simulink model "Full_Model_D_R6"  (R2013a)
settings: Solver=ode45  StartTime=0.0  StopTime=sim_length  MaxStep=1e-4  RelTol=1e-3
values from neighbouring files (symbols this model uses):
  A_Height_d = [1  0.02  0.00306066709295; 0  1  0.292172619905; 0  0  0.751477293075]    [Height_Controller_SS_D_Data.mat]    (also in Height_Controller_Sample_Time.m = A_d)
  A_Roll_d = [1  0.02  0.00957373027909; 0  1  0.913912481482; 0  0  0.751477293075]    [Roll_Controller_SS_D_Data.mat]    (also in Roll_Controller_Sample_Time.m = A_d)
  A_x_d = [1  0.725237004499; 0  0.506103765926]    [xy_Controller_PD_D_Data.mat]    (also in xy_Controller_PID_D_Data.mat; xy_Controller_Sample_Time.m = sys_d.a; xy_Controller_Sample_Time_2.m = sys_d.a)
  A_Yaw_d = [1  0.02  0.000714353321797; 0  1  0.0681924806681; 0  0  0.751477293075]    [Yaw_Controller_SS_D_Data.mat]    (also in Yaw_Controller_Sample_Time.m = A_d)
  B_Height_d = [0.000298297262238 0.0437238156136 0.248522706925]    [Height_Controller_SS_D_Data.mat]    (also in Height_Controller_Sample_Time.m = B_d)
  B_Roll_d = [0.000933070289885 0.136767575416 0.248522706925]    [Roll_Controller_SS_D_Data.mat]    (also in Roll_Controller_Sample_Time.m = B_d)
  B_x_d = [3.95796081795 7.11457501414]    [xy_Controller_PD_D_Data.mat]    (also in xy_Controller_PID_D_Data.mat; xy_Controller_Sample_Time.m = sys_d.b; xy_Controller_Sample_Time_2.m = sys_d.b)
  B_Yaw_d = [7.15569400366e-05 0.0103985455153 0.248522706925]    [Yaw_Controller_SS_D_Data.mat]    (also in Yaw_Controller_Sample_Time.m = B_d)
  C_Height_d = [1 0 0]    [Height_Controller_SS_D_Data.mat]    (also in Height_Controller_Sample_Time.m = C_d)
  C_Roll_d = [1  0  0; 0  1  0]    [Roll_Controller_SS_D_Data.mat]    (also in Roll_Controller_Sample_Time.m = C_d)
  C_x_d = [1 0]    [xy_Controller_PD_D_Data.mat]    (also in xy_Controller_PID_D_Data.mat; xy_Controller_Sample_Time.m = sys_d.c; xy_Controller_Sample_Time_2.m = sys_d.c)
  C_Yaw_d = [1  0  0; 0  1  0]    [Yaw_Controller_SS_D_Data.mat]    (also in Yaw_Controller_Sample_Time.m = C_d)
  coeff_speed1 = [-597.852411164 15567.4958959 -112629.522245 385376.825444 -722286.582234 762343.511164 -424427.181206 96698.0914793]    [Model_Parameters.mat]
  coeff_speed2 = [-33137.8630803 359389.817861 -1655728.0128 4197976.53355 -6322358.45977 5652250.74311 -2774846.33743 576528.840344]    [Model_Parameters.mat]
  coeff_speed3 = [-11936.4686056 137218.314774 -666283.661319 1770733.67902 -2780453.20018 2577948.57948 -1305141.01347 277978.291866]    [Model_Parameters.mat]
  coeff_speed4 = [-6669.45808334 79913.0612752 -401123.444791 1094619.31774 -1754742.75761 1652252.04897 -844945.337957 180729.993964]    [Model_Parameters.mat]
  coeff_thrust1 = [411.996230985 -4101.92524784 17203.3662669 -39329.1303747 52812.747408 -41528.8245566 17635.526271 -3103.13769268]    [Model_Parameters.mat]
  coeff_thrust2 = [3.52133616408 187.041584587 -1860.27738451 7135.94114535 -14212.0789042 15650.5208884 -9059.28758852 2154.75680942]    [Model_Parameters.mat]
  coeff_thrust3 = [-509.084474191 5539.72556164 -25664.1372161 65589.3028623 -99834.0669633 90481.3955019 -45198.9623282 9597.06354792]    [Model_Parameters.mat]
  coeff_thrust4 = [270.975135723 -2599.21496486 10453.4946669 -22770.946547 28872.4244579 -21147.1170047 8185.59308918 -1264.84197054]    [Model_Parameters.mat]
  Drag = 4.45306861536e-07    [Model_Parameters.mat]
  F_Roll_d = A_Roll_d-G_Roll_d*C_Roll_d    [Script_Controller_Sample_Time.m]    (also in Test_Controller_Sample_Time.m)
  F_yIntercept = -10.4432883127    [Model_Parameters.mat]
  Feed_Forward_Height_d = 2    [Height_Controller_SS_D_Data.mat]    (also in Height_Controller_Sample_Time.m)
  Feed_Forward_Roll_d = 0.125    [Roll_Controller_SS_D_Data.mat]    (also in Roll_Controller_Sample_Time.m)
  Feed_Forward_Yaw_d = 0    [Yaw_Controller_SS_D_Data.mat]    (also in Yaw_Controller_Sample_Time.m)
  g = 9.81    [Model_Parameters.mat]
  G_Height_d = [1.56504668046 34.0074022073 8.86962171802]    [Height_Controller_SS_D_Data.mat]    (also in Height_Controller_Sample_Time.m = place(A_d',C_d',P)')
  G_Roll_d = [0.251889913145  0.0200094814614; 0.229685260441  0.24715204306; -0.000711541775691  -9.30790483026e-05]    [Roll_Controller_SS_D_Data.mat]    (also in Roll_Controller_Sample_Time.m = place(A_d',C_d',P)')
  G_x_d = [-0.193896234074 0.15962315642]    [xy_Controller_PD_D_Data.mat]    (also in xy_Controller_PID_D_Data.mat; xy_Controller_Sample_Time.m = place(A_x_d',C_x_d',P)'; xy_Controller_Sample_Time_2.m = place(A_x_d',C_x_d',P)')
  G_Yaw_d = [0.242030648398  0.0200584166088; 0.0044560948779  0.235341919238; -0.000643549416335  -0.000818909263128]    [Yaw_Controller_SS_D_Data.mat]    (also in Yaw_Controller_Sample_Time.m = place(A_d',C_d',P)')
  I_Phi = 0.127422725814    [Model_Parameters.mat]
  I_Psi = 0.236966962973    [Model_Parameters.mat]
  I_Theta = 0.122104044652    [Model_Parameters.mat]
  J = 8e-08    [Model_Parameters.mat]
  K_Height_d = [2.7513802614 0.716922726377 0.637441613793]    [Height_Controller_SS_D_Data.mat]    (also in Height_Controller_Sample_Time.m = K_Height_Reg(1:end-1))
  K_Height_i = -2.03246593773    [Height_Controller_SS_D_Data.mat]    (also in Height_Controller_Sample_Time.m = K_Height_Reg(end))
  K_Roll_d = [2.67637429311 0.450684169535 1.07098831744]    [Roll_Controller_SS_D_Data.mat]    (also in Roll_Controller_Sample_Time.m = K_Roll_Reg(1:end-1))
  K_Roll_i = -2.24117965782    [Roll_Controller_SS_D_Data.mat]    (also in Roll_Controller_Sample_Time.m = K_Roll_Reg(end))
  K_Yaw_d = [1.55130112498 0.960619912039 0.23556072791]    [Yaw_Controller_SS_D_Data.mat]    (also in Yaw_Controller_Sample_Time.m = K_Yaw_Reg(1:end-1))
  K_Yaw_i = -1.12834490639    [Yaw_Controller_SS_D_Data.mat]    (also in Yaw_Controller_Sample_Time.m = K_Yaw_Reg(end))
  Kd_x = 0    [xy_Controller_PD_D_Data.mat]    (also in xy_Controller_PID_D_Data.mat = 0.0186150358972; xy_Controller_Sample_Time.m = get(C,'Kd'); xy_Controller_Sample_Time_2.m = get(C,'Kd'))
  Kd_y = 0    [xy_Controller_PD_D_Data.mat]    (also in xy_Controller_PID_D_Data.mat = 0.0186150358972; xy_Controller_Sample_Time.m = Kd_x; xy_Controller_Sample_Time_2.m = Kd_x)
  Kf = 9.48907430341    [Model_Parameters.mat]
  Ki_x = 0.000229999504243    [xy_Controller_PD_D_Data.mat]    (also in xy_Controller_PID_D_Data.mat = 0.000234605659833; xy_Controller_Sample_Time.m = get(C,'Ki'); xy_Controller_Sample_Time_2.m = get(C,'Ki'))
  Ki_y = 0.000229999504243    [xy_Controller_PD_D_Data.mat]    (also in xy_Controller_PID_D_Data.mat = 0.000234605659833; xy_Controller_Sample_Time.m = Ki_x; xy_Controller_Sample_Time_2.m = Ki_x)
  Kp_x = 0.032529495388    [xy_Controller_PD_D_Data.mat]    (also in xy_Controller_PID_D_Data.mat = 0.0333125747447; xy_Controller_Sample_Time.m = get(C,'Kp'); xy_Controller_Sample_Time_2.m = get(C,'Kp'))
  Kp_y = 0.032529495388    [xy_Controller_PD_D_Data.mat]    (also in xy_Controller_PID_D_Data.mat = 0.0333125747447; xy_Controller_Sample_Time.m = Kp_x; xy_Controller_Sample_Time_2.m = Kp_x)
  Kw = 501.513336009    [Model_Parameters.mat]
  L = 0.338    [Model_Parameters.mat]
  Mass = 2.26    [Model_Parameters.mat]
  Motor_TimeConstant = 0.07    [Model_Parameters.mat]
  NoiseDelay = 0    [All_Controller_Sample_Time.m]
  NoiseMean = 0    [All_Controller_Sample_Time.m]
  omega_0 = (0-F_yIntercept)/Kf    [Test_Controller_Sample_Time.m]    (also in Yaw_Controller_Sample_Time.m = 520)
  omega_Lim = (0-F_yIntercept)/Kf    [Test_Controller_Sample_Time.m]
  Phi_IC = (0/180)*pi    (= 0)    [Test_Controller_Sample_Time.m]
  Pitch_Setpoint = 0    [Test_Controller_Sample_Time.m]
  PropDelay = 0    [All_Controller_Sample_Time.m]
  Psi_IC = (0/180)*pi    (= 0)    [Test_Controller_Sample_Time.m]
  PWM_LimHigher = 2    [Test_Controller_Sample_Time.m]
  PWM_LimLower = 1.1    [Test_Controller_Sample_Time.m]
  Speed_yIntercept = -347.939581678    [Model_Parameters.mat]
  Tau_filter1 = 0.5    [All_Controller_Sample_Time.m]
  Theta_IC = (5/180)*pi    (= 0.0872664625997)    [Test_Controller_Sample_Time.m]
  Ts = 20e-3    (= 0.02)    [All_Controller_Sample_Time.m]
  Ts2 = 1    [All_Controller_Sample_Time.m]
  ViscousDamping = 36*sin(20/180*pi)/8    [All_Controller_Sample_Time.m]
  Yaw_Setpoint = 0    [Test_Controller_Sample_Time.m]
undefined symbols (not defined in the file or in its folder): DiscIntNeverNeededParam
libraries: simulink x9, commnoisgen2 x7
(part 1 of 2)
settings Model: Creator=Ross  LastModifiedBy=Ross

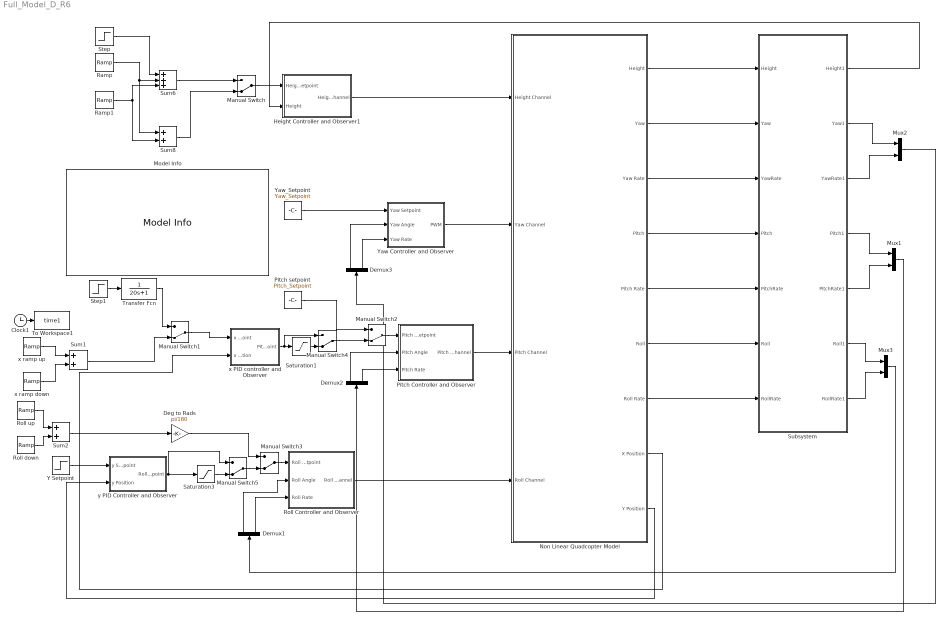
== system Full_Model_D_R6 ==
  Clock1 : Clock
  Deg to Rads : Gain  Gain=pi/180  SampleTime=Ts
  Demux1 : Demux  Outputs=2
  Demux2 : Demux  Outputs=2
  Demux3 : Demux  Outputs=2
  Height Controller and Observer1 : Subsystem
  Manual Switch{,1..5} (6 alike) : ManualSwitch  CurrentSetting=0
  Model Info : simulink/Model-Wide Utilities/Model Info  InitialBlockCM=None  BlockCM=None  Frame=on  DisplayStringWithTags=|  HorizontalTextAlignment=Center  LeftAlignmentValue=0.5  SourceBlockDiagram=Full_Model_D_R6  TagMaxNumber=20
      | %<ModelName>
      | Simulink Diagram Used in Testing of Controllers designed for Quadcopters
      | Model version is %<ModelVersion>
      | 
      | %<Created>
      | %<ModifiedBy>
      | %<ModifiedDate>
      | %<ModifiedComment>
      | 
      | 
      | %<LastModifiedBy>
      | %<LastModificationDate>
      | %<Description>
  Mux1 : Mux  Inputs=2
  Mux2 : Mux  Inputs=2
  Mux3 : Mux  Inputs=2
  Non Linear Quadcopter Model : Subsystem
  Pitch Controller and Observer : Subsystem
  Pitch setpoint : Constant  Value=Pitch_Setpoint
  Ramp : simulink/Sources/Ramp  slope=1  start=5  X0=0
  Ramp1 : simulink/Sources/Ramp  slope=-1  start=10  X0=0
  Roll Controller and Observer : Subsystem
  Roll down : simulink/Sources/Ramp  slope=-20  start=30  X0=0
  Roll up : simulink/Sources/Ramp  slope=20  start=20  X0=0
  Saturation1 : Saturate  UpperLimit=(30/180)*pi  LowerLimit=-(30/180)*pi
  Saturation3 : Saturate  UpperLimit=(30/180)*pi  LowerLimit=-(30/180)*pi
  Step : Step  Time=15  After=2  SampleTime=0
  Step1 : Step  Time=20  After=5  SampleTime=0
  Subsystem : Subsystem
  Sum1 : Sum
  Sum2 : Sum
  Sum6 : Sum  Inputs=+++
  Sum8 : Sum
  To Workspace1 : ToWorkspace  VariableName=time1  SampleTime=Ts  SaveFormat=Timeseries
  Transfer Fcn : TransferFcn  Denominator=[20 1]
  Y Setpoint : Step  Time=50  After=5  SampleTime=0
  Yaw Controller and Observer : Subsystem
  Yaw_Setpoint : Constant  Value=Yaw_Setpoint
  x PID controller and Observer : Subsystem
  x ramp down : simulink/Sources/Ramp  slope=-2  start=30  X0=0
  x ramp up : simulink/Sources/Ramp  slope=2  start=20  X0=0
  y PID Controller and Observer : Subsystem
  wires:
  Ramp/1 -> Sum8/1, Sum6/2
  Ramp1/1 -> Sum8/2, Sum6/3
  Step/1 -> Sum6/1
  Manual Switch/1 -> Height Controller and Observer1/1(Height Setpoint)
  Sum8/1 -> Manual Switch/2
  Sum6/1 -> Manual Switch/1
  Yaw_Setpoint/1 -> Yaw Controller and Observer/1(Yaw Setpoint)
  Pitch Controller and Observer/1(Pitch Channel) -> Non Linear Quadcopter Model/3(Pitch Channel)
  Yaw Controller and Observer/1(PWM) -> Non Linear Quadcopter Model/2(Yaw Channel)
  Height Controller and Observer1/1(Height Channel) -> Non Linear Quadcopter Model/1(Height Channel)
  Roll Controller and Observer/1(Roll Channel) -> Non Linear Quadcopter Model/4(Roll Channel)
  Non Linear Quadcopter Model/1(Height) -> Subsystem/1(Height)
  Non Linear Quadcopter Model/2(Yaw) -> Subsystem/2(Yaw)
  Non Linear Quadcopter Model/3(Yaw Rate) -> Subsystem/3(YawRate)
  Non Linear Quadcopter Model/4(Pitch) -> Subsystem/4(Pitch)
  Non Linear Quadcopter Model/5(Pitch Rate) -> Subsystem/5(PitchRate)
  Non Linear Quadcopter Model/7(Roll Rate) -> Subsystem/7(RollRate)
  Subsystem/1(Height1) -> Height Controller and Observer1/2(Height)
  Subsystem/2(Yaw1) -> Mux2/1
  Subsystem/3(YawRate1) -> Mux2/2
  Subsystem/4(Pitch1) -> Mux1/1
  Subsystem/5(PitchRate1) -> Mux1/2
  Subsystem/6("Roll1 ") -> Mux3/1
  Subsystem/7(RollRate1) -> Mux3/2
  Non Linear Quadcopter Model/9(Y Position) -> y PID Controller and Observer/2(y Position)
  Clock1/1 -> To Workspace1/1
  Non Linear Quadcopter Model/8(X Position) -> x PID controller and Observer/2(x Position)
  x ramp up/1 -> Sum1/1
  x ramp down/1 -> Sum1/2
  Sum1/1 -> Manual Switch1/2
  Mux2/1 -> Demux3/1
  Demux3/2 -> Yaw Controller and Observer/3(Yaw Rate)
  Demux3/1 -> Yaw Controller and Observer/2(Yaw Angle)
  Mux1/1 -> Demux2/1
  Demux2/2 -> Pitch Controller and Observer/3(Pitch Rate)
  Demux2/1 -> Pitch Controller and Observer/2(Pitch Angle)
  Mux3/1 -> Demux1/1
  Demux1/2 -> Roll Controller and Observer/3(Roll Rate)
  Demux1/1 -> Roll Controller and Observer/2(Roll Angle)
  Manual Switch2/1 -> Pitch Controller and Observer/1(Pitch Setpoint)
  Pitch setpoint/1 -> Manual Switch2/1
  Manual Switch3/1 -> Roll Controller and Observer/1(Roll Setpoint)
  y PID Controller and Observer/1(Roll Setpoint) -> Manual Switch5/1, Saturation3/1
  x PID controller and Observer/1(Pitch Setpoint) -> Manual Switch4/1, Saturation1/1
  Manual Switch1/1 -> x PID controller and Observer/1(x Setpoint)
  Step1/1 -> Transfer Fcn/1
  Saturation1/1 -> Manual Switch4/2
  Saturation3/1 -> Manual Switch5/2
  Manual Switch4/1 -> Manual Switch2/2
  Manual Switch5/1 -> Manual Switch3/2
  Transfer Fcn/1 -> Manual Switch1/1
  Non Linear Quadcopter Model/6(Roll) -> Subsystem/6(Roll)
  Deg to Rads/1 -> Manual Switch3/1
  Roll down/1 -> Sum2/2
  Roll up/1 -> Sum2/1
  Sum2/1 -> Deg to Rads/1
  Y Setpoint/1 -> y PID Controller and Observer/1(y Setpoint)

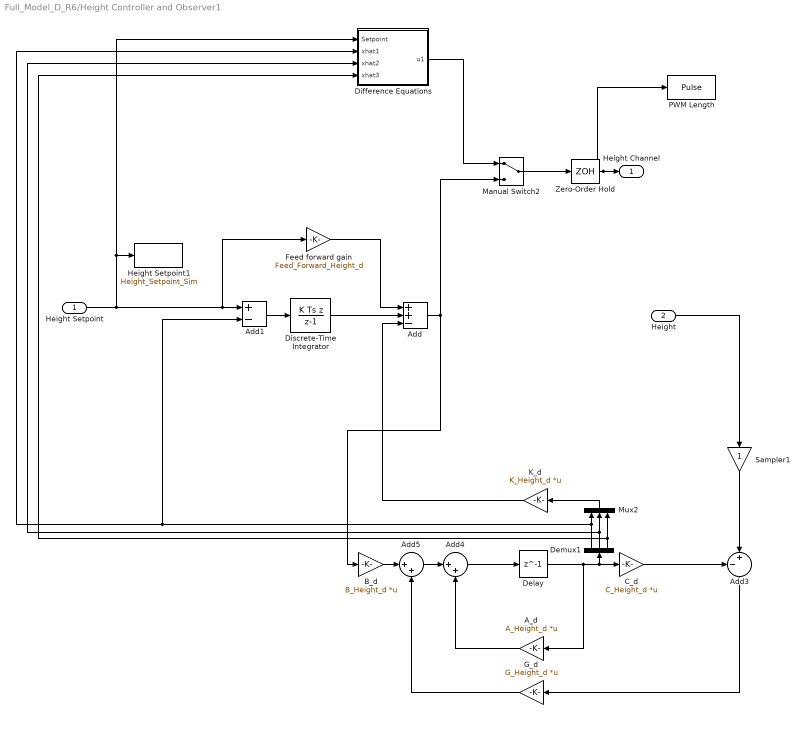
== system Full_Model_D_R6/Height Controller and Observer1 ==
  Height Setpoint : Inport
  Height : Inport  Port=2
  A_d : Gain  Gain=A_Height_d  Multiplication=Matrix(K*u)  SampleTime=Ts
  Add : Sum  Inputs=++-
  Add1 : Sum  Inputs=+-
  Add3 : Sum  Inputs=-+|
  Add4 : Sum  Inputs=|++
  Add5 : Sum  Inputs=|++
  "B_d " : Gain  Gain=B_Height_d  Multiplication=Matrix(K*u)  SampleTime=Ts
  "C_d " : Gain  Gain=C_Height_d  Multiplication=Matrix(K*u)  SampleTime=Ts
  Delay : Delay  DelayLength=1  InitialCondition=0  SampleTime=Ts
  Demux1 : Demux  Outputs=3
  Difference Equations : Subsystem
  Discrete-Time Integrator : DiscreteIntegrator  IntegratorMethod=Integration: Backward Euler  gainval=-K_Height_i  SampleTime=Ts  ICPrevOutput=DiscIntNeverNeededParam  ICPrevScaledInput=DiscIntNeverNeededParam
  Feed forward gain : Gain  Gain=Feed_Forward_Height_d  SampleTime=Ts
  G_d : Gain  Gain=G_Height_d  Multiplication=Matrix(K*u)  SampleTime=Ts
  Height Setpoint1 : ToWorkspace  VariableName=Height_Setpoint_Sim  SampleTime=-1  SaveFormat=Timeseries
  K_d : Gain  Gain=K_Height_d  Multiplication=Matrix(K*u)  SampleTime=Ts
  Manual Switch2 : ManualSwitch
  Mux2 : Mux  Inputs=3
  PWM Length : ToWorkspace  VariableName=Pulse  SampleTime=-1  SaveFormat=Timeseries
  Sampler1 : Gain  SampleTime=Ts
  Zero-Order Hold : ZeroOrderHold  SampleTime=Ts
  Height Channel : Outport
  wires:
  Add/1 -> Manual Switch2/2, "B_d "/1
  "B_d "/1 -> Add5/1
  K_d/1 -> Add/3
  Demux1/2 -> Difference Equations/3(xhat2), Mux2/2
  Sampler1/1 -> Add3/2
  Add4/1 -> Delay/1
  Add3/1 -> G_d/1
  Demux1/3 -> Mux2/3, Difference Equations/4(xhat3)
  Demux1/1 -> Difference Equations/2(xhat1), Add1/2, Mux2/1
  G_d/1 -> Add5/2
  Delay/1 -> Demux1/1, "C_d "/1, A_d/1
  Mux2/1 -> K_d/1
  "C_d "/1 -> Add3/1
  A_d/1 -> Add4/2
  Add5/1 -> Add4/1
  Height/1 -> Sampler1/1
  Height Setpoint/1 -> Difference Equations/1(Setpoint), Height Setpoint1/1, Feed forward gain/1, Add1/1
  Zero-Order Hold/1 -> PWM Length/1, Height Channel/1
  Feed forward gain/1 -> Add/1
  Add1/1 -> Discrete-Time Integrator/1
  Discrete-Time Integrator/1 -> Add/2
  Manual Switch2/1 -> Zero-Order Hold/1
  Difference Equations/1(u1) -> Manual Switch2/1

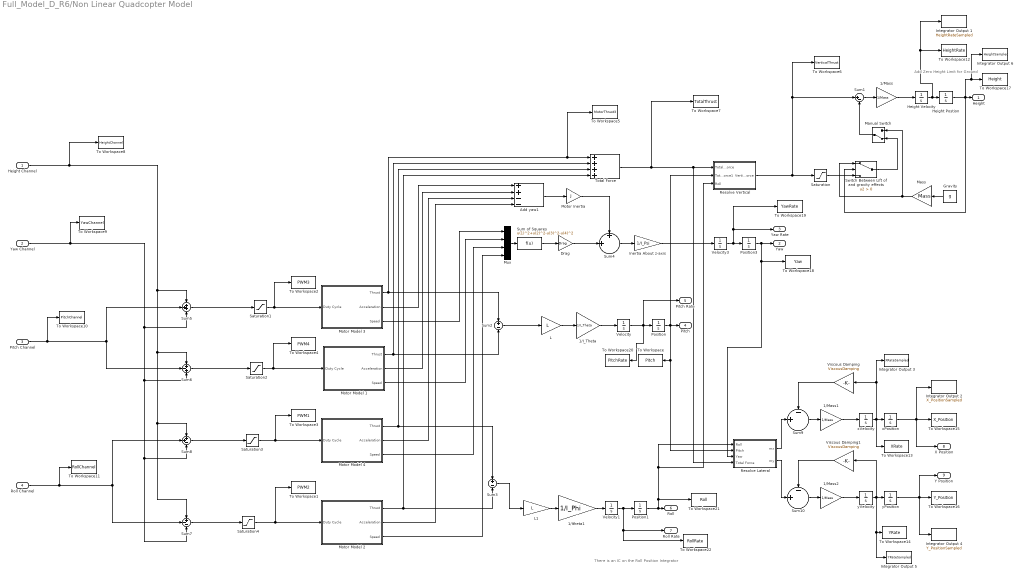
== system Full_Model_D_R6/Non Linear Quadcopter Model ==
  note: There is an IC on the Roll
      | Position Integrator
  note: Add Zero Height Limit
      | for Ground
  Height Channel : Inport
  Yaw Channel : Inport  Port=2
  Pitch Channel : Inport  Port=3
  Roll Channel : Inport  Port=4
  1/I_Theta : Gain  Gain=1/I_Theta
  1/Itheta1 : Gain  Gain=1/I_Phi
  1/Mass : Gain  Gain=1/Mass
  1/Mass1 : Gain  Gain=1/Mass
  1/Mass2 : Gain  Gain=1/Mass
  Add yaw1 : Sum  Inputs=++--
  Drag : Gain  Gain=Drag
  Gravity : Constant  Value=g
  Height Postion : Integrator  LowerSaturationLimit=0
  Height Velocity : Integrator
  Inertia About z-axis : Gain  Gain=1/I_Psi
  Integrator Output 1 : ToWorkspace  VariableName=HeightRateSampled  SampleTime=Ts  SaveFormat=Timeseries
  Integrator Output 2 : ToWorkspace  VariableName=X_PositionSampled  SampleTime=Ts  SaveFormat=Timeseries
  Integrator Output 3 : ToWorkspace  VariableName=XRateSampled  SampleTime=Ts  SaveFormat=Timeseries
  Integrator Output 4 : ToWorkspace  VariableName=Y_PositionSampled  SampleTime=Ts  SaveFormat=Timeseries
  Integrator Output 5 : ToWorkspace  VariableName=YRateSampled  SampleTime=Ts  SaveFormat=Timeseries
  Integrator Output 6 : ToWorkspace  VariableName=HeightSampled  SampleTime=Ts  SaveFormat=Timeseries
  L : Gain  Gain=L
  L1 : Gain  Gain=L
  Manual Switch : ManualSwitch  CurrentSetting=0
  Mass : Gain  Gain=Mass
  Motor Inertia : Gain  Gain=J
  Motor Model 1 : Subsystem
  Motor Model 2 : Subsystem
  Motor Model 3 : Subsystem
  Motor Model 4 : Subsystem
  Mux : Mux
  Position : Integrator  InitialCondition=Theta_IC
  Position1 : Integrator  InitialCondition=Phi_IC
  Position3 : Integrator  InitialCondition=Psi_IC
  Resolve Lateral : Subsystem
  Resolve Vertical : Subsystem
  Saturation : Saturate  UpperLimit=Mass*g  LowerLimit=-inf
  Saturation{1..4} (4 alike) : Saturate  UpperLimit=PWM_LimHigher  LowerLimit=PWM_LimLower
  Sum of Squares : Fcn  Expr=u(1)^2+u(2)^2-u(3)^2-u(4)^2
  Sum1 : Sum  Inputs=|+-
  Sum10 : Sum  Inputs=-|||+||||
  Sum2 : Sum  Inputs=+|-
  Sum3 : Sum  Inputs=+|-
  Sum4 : Sum  Inputs=+|||+||||
  Sum5 : Sum  Inputs=+++
  Sum6 : Sum  Inputs=+-+
  Sum7 : Sum  Inputs=+--
  Sum8 : Sum  Inputs=++-
  Sum9 : Sum  Inputs=-|||+||||
  Switch Between Lift of and gravity effects : Switch  Criteria=u2 > Threshold
  To Workspace : ToWorkspace  VariableName=Pitch  SampleTime=-1  SaveFormat=Timeseries
  To Workspace1 : ToWorkspace  VariableName=PWM2  SampleTime=-1  SaveFormat=Timeseries
  To Workspace10 : ToWorkspace  VariableName=PitchChannel  SampleTime=-1  SaveFormat=Timeseries
  To Workspace11 : ToWorkspace  VariableName=RollChannel  SampleTime=-1  SaveFormat=Timeseries
  To Workspace12 : ToWorkspace  VariableName=HeightRate  SampleTime=-1  SaveFormat=Timeseries
  To Workspace13 : ToWorkspace  VariableName=XRate  SampleTime=-1  SaveFormat=Timeseries
  To Workspace14 : ToWorkspace  VariableName=YRate  SampleTime=-1  SaveFormat=Timeseries
  To Workspace15 : ToWorkspace  VariableName=X_Position  SampleTime=-1  SaveFormat=Timeseries
  To Workspace16 : ToWorkspace  VariableName=Y_Position  SampleTime=-1  SaveFormat=Timeseries
  To Workspace17 : ToWorkspace  VariableName=Height  SampleTime=-1  SaveFormat=Timeseries
  To Workspace18 : ToWorkspace  VariableName=Yaw  SampleTime=-1  SaveFormat=Timeseries
  To Workspace19 : ToWorkspace  VariableName=YawRate  SampleTime=-1  SaveFormat=Timeseries
  To Workspace2 : ToWorkspace  VariableName=PWM3  SampleTime=-1  SaveFormat=Timeseries
  To Workspace20 : ToWorkspace  VariableName=PitchRate  SampleTime=-1  SaveFormat=Timeseries
  To Workspace21 : ToWorkspace  VariableName=Roll  SampleTime=-1  SaveFormat=Timeseries
  To Workspace22 : ToWorkspace  VariableName=RollRate  SampleTime=-1  SaveFormat=Timeseries
  To Workspace3 : ToWorkspace  VariableName=PWM1  SampleTime=-1  SaveFormat=Timeseries
  To Workspace4 : ToWorkspace  VariableName=PWM4  SampleTime=-1  SaveFormat=Timeseries
  To Workspace5 : ToWorkspace  VariableName=MotorThrust3  SampleTime=-1  SaveFormat=Timeseries
  To Workspace6 : ToWorkspace  VariableName=VerticalThrust  SampleTime=-1  SaveFormat=Timeseries
  To Workspace7 : ToWorkspace  VariableName=TotalThrust  SampleTime=-1  SaveFormat=Timeseries
  To Workspace8 : ToWorkspace  VariableName=HeightChannel  SampleTime=-1  SaveFormat=Timeseries
  To Workspace9 : ToWorkspace  VariableName=YawChannel  SampleTime=-1  SaveFormat=Timeseries
  Total Force : Sum  Inputs=++++
  Velocity : Integrator
  Velocity1 : Integrator
  Velocity3 : Integrator
  Viscous Damping : Gain  Gain=ViscousDamping
  Viscous Damping1 : Gain  Gain=ViscousDamping
  xPosition : Integrator
  xVelocity : Integrator
  yPosition : Integrator
  yVelocity : Integrator
  Height : Outport
  Yaw : Outport  Port=2
  Yaw Rate : Outport  Port=3
  Pitch : Outport  Port=4
  Pitch Rate : Outport  Port=5
  Roll : Outport  Port=6
  Roll Rate : Outport  Port=7
  X Position : Outport  Port=8
  Y Position : Outport  Port=9
  wires:
  Sum1/1 -> 1/Mass/1
  Pitch Channel/1 -> Sum6/2, Sum5/2, To Workspace10/1
  Add yaw1/1 -> Motor Inertia/1
  1/Mass/1 -> Height Velocity/1
  Motor Inertia/1 -> Sum4/1
  1/Mass1/1 -> xVelocity/1
  Sum9/1 -> 1/Mass1/1
  Viscous Damping/1 -> Sum9/1
  xVelocity/1 -> To Workspace13/1, Viscous Damping/1, Integrator Output 3/1, xPosition/1
  Motor Model 3/2(Acceleration) -> Add yaw1/1
  Sum8/1 -> Saturation3/1
  Sum2/1 -> L/1
  1/I_Theta/1 -> Velocity/1
  Velocity/1 -> To Workspace20/1, Pitch Rate/1, Position/1
  Position/1 -> Resolve Vertical/2(Total Force1), Pitch/1, Resolve Lateral/2(Pitch), To Workspace/1
  Total Force/1 -> To Workspace7/1, Resolve Lateral/4(Total Force), Resolve Vertical/1(Total Force)
  Sum of Squares/1 -> Drag/1
  Drag/1 -> Sum4/2
  Position3/1 -> Resolve Lateral/3(Yaw), To Workspace18/1, Yaw/1
  Velocity3/1 -> To Workspace19/1, Yaw Rate/1, Position3/1
  Inertia About z-axis/1 -> Velocity3/1
  Motor Model 2/1(Thrust) -> Total Force/4, Sum3/2
  L1/1 -> 1/Itheta1/1
  Velocity1/1 -> To Workspace22/1, Roll Rate/1, Position1/1
  Sum3/1 -> L1/1
  Position1/1 -> Roll/1, To Workspace21/1, Resolve Lateral/1(Roll), Resolve Vertical/3(Roll)
  1/Itheta1/1 -> Velocity1/1
  Motor Model 3/1(Thrust) -> To Workspace5/1, Total Force/1, Sum2/1
  Sum10/1 -> 1/Mass2/1
  1/Mass2/1 -> yVelocity/1
  Viscous Damping1/1 -> Sum10/1
  yVelocity/1 -> Viscous Damping1/1, Integrator Output 5/1, To Workspace14/1, yPosition/1
  Sum7/1 -> Saturation4/1
  Motor Model 4/2(Acceleration) -> Add yaw1/3
  Motor Model 1/1(Thrust) -> Total Force/2, Sum2/2
  Sum4/1 -> Inertia About z-axis/1
  Motor Model 4/1(Thrust) -> Total Force/3, Sum3/1
  Height Channel/1 -> To Workspace8/1, Sum6/1, Sum7/1, Sum8/1, Sum5/1
  Yaw Channel/1 -> To Workspace9/1, Sum7/3, Sum8/3, Sum6/3, Sum5/3
  Motor Model 1/2(Acceleration) -> Add yaw1/2
  Motor Model 2/2(Acceleration) -> Add yaw1/4
  Sum5/1 -> Saturation1/1
  Roll Channel/1 -> To Workspace11/1, Sum8/2, Sum7/2
  Gravity/1 -> Mass/1
  Resolve Lateral/1(mx) -> Sum9/2
  Resolve Lateral/2(my) -> Sum10/2
  Motor Model 3/3(Speed) -> Mux/1
  Motor Model 1/3(Speed) -> Mux/2
  Motor Model 4/3(Speed) -> Mux/3
  Motor Model 2/3(Speed) -> Mux/4
  Mux/1 -> Sum of Squares/1
  L/1 -> 1/I_Theta/1
  Switch Between Lift of and gravity effects/1 -> Manual Switch/2
  Saturation/1 -> Switch Between Lift of and gravity effects/3
  Mass/1 -> Manual Switch/1, Switch Between Lift of and gravity effects/1
  Sum6/1 -> Saturation2/1
  Manual Switch/1 -> Sum1/2
  Resolve Vertical/1(Vertical Force) -> Sum1/1, To Workspace6/1, Saturation/1
  yPosition/1 -> Y Position/1, Integrator Output 4/1, To Workspace16/1
  Saturation1/1 -> Motor Model 3/1(Duty Cycle), To Workspace2/1
  Saturation2/1 -> Motor Model 1/1(Duty Cycle), To Workspace4/1
  Saturation3/1 -> Motor Model 4/1(Duty Cycle), To Workspace3/1
  Saturation4/1 -> Motor Model 2/1(Duty Cycle), To Workspace1/1
  Height Velocity/1 -> Integrator Output 1/1, To Workspace12/1, Height Postion/1
  xPosition/1 -> X Position/1, Integrator Output 2/1, To Workspace15/1
  Height Postion/1 -> Switch Between Lift of and gravity effects/2, Integrator Output 6/1, To Workspace17/1, Height/1

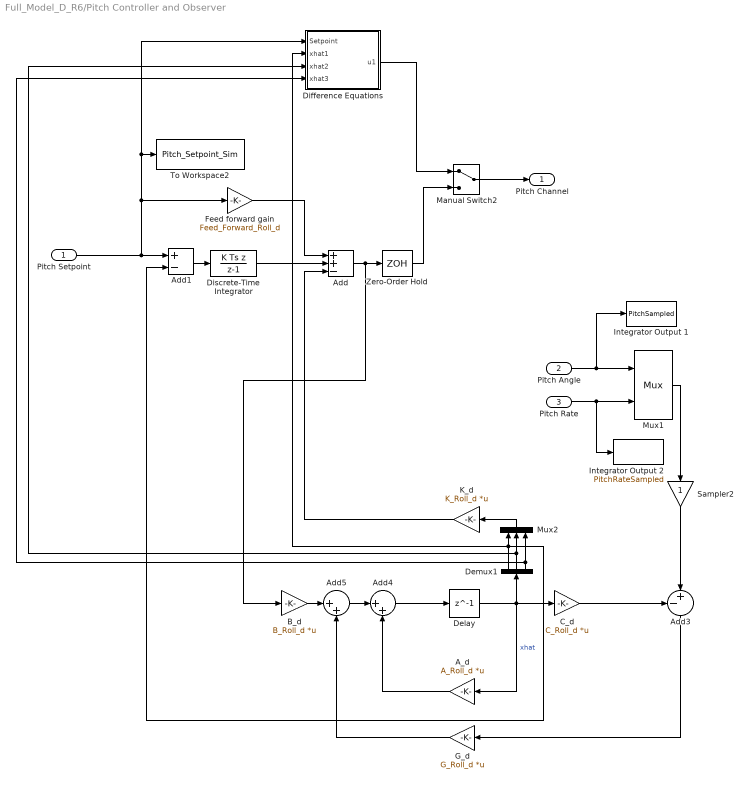
== system Full_Model_D_R6/Pitch Controller and Observer ==
  Pitch Setpoint : Inport
  Pitch Angle : Inport  Port=2
  Pitch Rate : Inport  Port=3
  A_d : Gain  Gain=A_Roll_d  Multiplication=Matrix(K*u)  SampleTime=Ts
  Add : Sum  Inputs=++-
  Add1 : Sum  Inputs=+-
  Add3 : Sum  Inputs=-+|
  Add4 : Sum  Inputs=|++
  Add5 : Sum  Inputs=|++
  "B_d " : Gain  Gain=B_Roll_d  Multiplication=Matrix(K*u)  SampleTime=Ts
  "C_d " : Gain  Gain=C_Roll_d  Multiplication=Matrix(K*u)  SampleTime=Ts
  Delay : Delay  DelayLength=1  InitialCondition=0  SampleTime=Ts
  Demux1 : Demux  Outputs=3
  Difference Equations : Subsystem
  Discrete-Time Integrator : DiscreteIntegrator  IntegratorMethod=Integration: Backward Euler  gainval=-K_Roll_i  SampleTime=Ts  ICPrevOutput=DiscIntNeverNeededParam  ICPrevScaledInput=DiscIntNeverNeededParam
  Feed forward gain : Gain  Gain=Feed_Forward_Roll_d  SampleTime=Ts
  G_d : Gain  Gain=G_Roll_d  Multiplication=Matrix(K*u)  SampleTime=Ts
  Integrator Output 1 : ToWorkspace  VariableName=PitchSampled  SampleTime=Ts  SaveFormat=Timeseries
  Integrator Output 2 : ToWorkspace  VariableName=PitchRateSampled  SampleTime=Ts  SaveFormat=Timeseries
  K_d : Gain  Gain=K_Roll_d  Multiplication=Matrix(K*u)  SampleTime=Ts
  Manual Switch2 : ManualSwitch
  Mux1 : Mux  Inputs=2
      settings: DisplayOption=signals
  Mux2 : Mux  Inputs=3
  Sampler2 : Gain  SampleTime=Ts
  To Workspace2 : ToWorkspace  VariableName=Pitch_Setpoint_Sim  SampleTime=-1  SaveFormat=Timeseries
  Zero-Order Hold : ZeroOrderHold  SampleTime=Ts
  Pitch Channel : Outport
  wires:
  Add5/1 -> Add4/1
  Demux1/3 -> Difference Equations/4(xhat3), Mux2/3
  Mux1/1 -> Sampler2/1
  G_d/1 -> Add5/2
  Demux1/2 -> Difference Equations/3(xhat2), Mux2/2
  A_d/1 -> Add4/2
  Add4/1 -> Delay/1
  "C_d "/1 -> Add3/1
  K_d/1 -> Add/3
  Sampler2/1 -> Add3/2
  Add/1 -> "B_d "/1, Zero-Order Hold/1
  "B_d "/1 -> Add5/1
  Mux2/1 -> K_d/1
  Add3/1 -> G_d/1
  Delay/1 -> "C_d "/1, Demux1/1, A_d/1  "xhat"
  Zero-Order Hold/1 -> Manual Switch2/2
  Discrete-Time Integrator/1 -> Add/2
  Pitch Setpoint/1 -> To Workspace2/1, Difference Equations/1(Setpoint), Feed forward gain/1, Add1/1
  Add1/1 -> Discrete-Time Integrator/1
  Feed forward gain/1 -> Add/1
  Pitch Angle/1 -> Integrator Output 1/1, Mux1/1
  Pitch Rate/1 -> Integrator Output 2/1, Mux1/2
  Difference Equations/1(u1) -> Manual Switch2/1
  Manual Switch2/1 -> Pitch Channel/1
  Demux1/1 -> Difference Equations/2(xhat1), Add1/2, Mux2/1

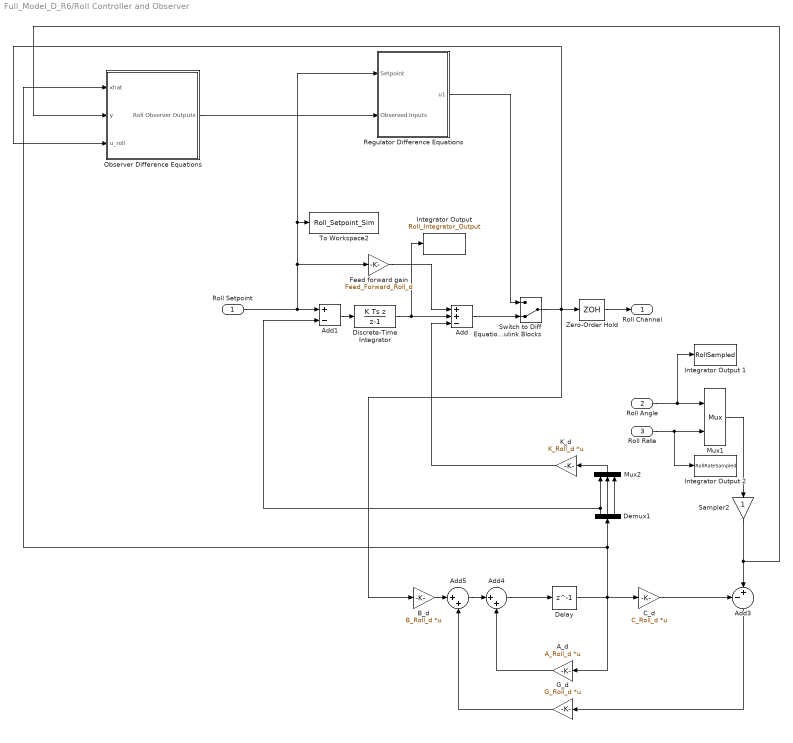
== system Full_Model_D_R6/Roll Controller and Observer ==
  Roll Setpoint : Inport
  Roll Angle : Inport  Port=2
  Roll Rate : Inport  Port=3
  A_d : Gain  Gain=A_Roll_d  Multiplication=Matrix(K*u)  SampleTime=Ts
  Add : Sum  Inputs=++-
  Add1 : Sum  Inputs=+-  SampleTime=Ts
  Add3 : Sum  Inputs=-+|
  Add4 : Sum  Inputs=|++
  Add5 : Sum  Inputs=|++
  "B_d " : Gain  Gain=B_Roll_d  Multiplication=Matrix(K*u)  SampleTime=Ts
  "C_d " : Gain  Gain=C_Roll_d  Multiplication=Matrix(K*u)  SampleTime=Ts
  Delay : Delay  DelayLength=1  InitialCondition=0  SampleTime=Ts
  Demux1 : Demux  Outputs=3
  Discrete-Time Integrator : DiscreteIntegrator  IntegratorMethod=Integration: Backward Euler  gainval=-K_Roll_i  SampleTime=Ts  ICPrevOutput=DiscIntNeverNeededParam  ICPrevScaledInput=DiscIntNeverNeededParam
  Feed forward gain : Gain  Gain=Feed_Forward_Roll_d  SampleTime=Ts
  G_d : Gain  Gain=G_Roll_d  Multiplication=Matrix(K*u)  SampleTime=Ts
  "Integrator Output " : ToWorkspace  VariableName=Roll_Integrator_Output  SampleTime=-1  SaveFormat=Timeseries
  Integrator Output 1 : ToWorkspace  VariableName=RollSampled  SampleTime=Ts  SaveFormat=Timeseries
  Integrator Output 2 : ToWorkspace  VariableName=RollRateSampled  SampleTime=Ts  SaveFormat=Timeseries
  K_d : Gain  Gain=K_Roll_d  Multiplication=Matrix(K*u)  SampleTime=Ts
  Mux1 : Mux  Inputs=2
      settings: DisplayOption=signals
  Mux2 : Mux  Inputs=3
  Observer Difference Equations : Subsystem
  Regulator Difference Equations : Subsystem
  Sampler2 : Gain  SampleTime=Ts
  Switch to Diff Equations From Simulink Blocks : ManualSwitch  CurrentSetting=0
  To Workspace2 : ToWorkspace  VariableName=Roll_Setpoint_Sim  SampleTime=-1  SaveFormat=Timeseries
  Zero-Order Hold : ZeroOrderHold  SampleTime=Ts
  Roll Channel : Outport
  wires:
  Add5/1 -> Add4/1
  Demux1/3 -> Mux2/3
  Mux1/1 -> Sampler2/1
  G_d/1 -> Add5/2
  A_d/1 -> Add4/2
  Add4/1 -> Delay/1
  "C_d "/1 -> Add3/1
  K_d/1 -> Add/3
  Sampler2/1 -> Observer Difference Equations/2(y), Add3/2
  "B_d "/1 -> Add5/1
  Mux2/1 -> K_d/1
  Add3/1 -> G_d/1
  Discrete-Time Integrator/1 -> "Integrator Output "/1, Add/2
  Add1/1 -> Discrete-Time Integrator/1
  Feed forward gain/1 -> Add/1
  Demux1/2 -> Mux2/2
  Roll Setpoint/1 -> Regulator Difference Equations/1(Setpoint), To Workspace2/1, Feed forward gain/1, Add1/1
  Regulator Difference Equations/1(u1) -> Switch to Diff Equations From Simulink Blocks/1
  Zero-Order Hold/1 -> Roll Channel/1
  Roll Angle/1 -> Integrator Output 1/1, Mux1/1
  Roll Rate/1 -> Integrator Output 2/1, Mux1/2
  Delay/1 -> Observer Difference Equations/1(xhat), Demux1/1, A_d/1, "C_d "/1
  Add/1 -> Switch to Diff Equations From Simulink Blocks/2
  Demux1/1 -> Add1/2, Mux2/1
  Observer Difference Equations/1(Roll Observer Outputs) -> Regulator Difference Equations/2(Observed Inputs)
  Switch to Diff Equations From Simulink Blocks/1 -> "B_d "/1, Observer Difference Equations/3(u_roll), Zero-Order Hold/1

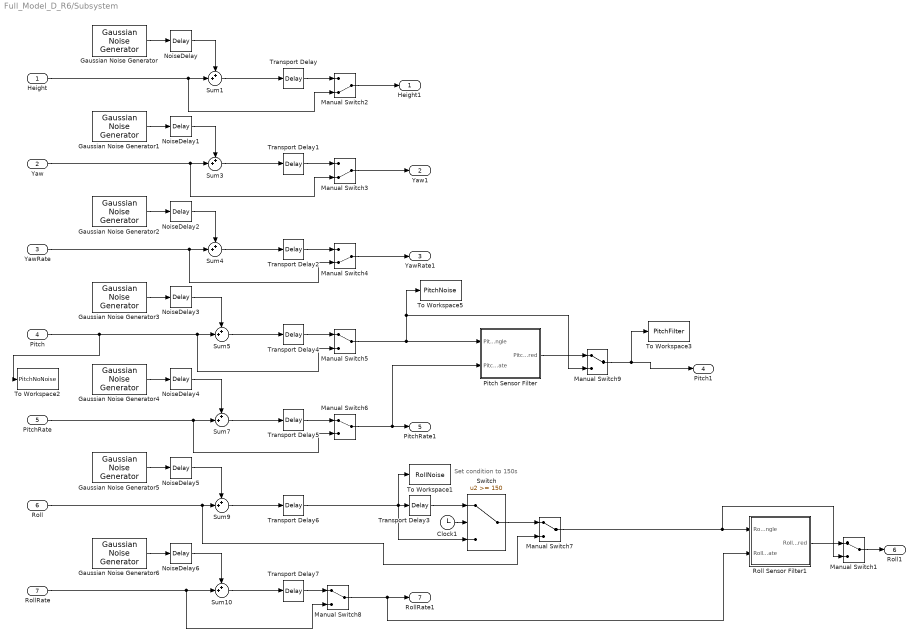
== system Full_Model_D_R6/Subsystem ==
  note: Set condition to 150s
  Height : Inport
  Yaw : Inport  Port=2
  YawRate : Inport  Port=3
  Pitch : Inport  Port=4
  PitchRate : Inport  Port=5
  Roll : Inport  Port=6
  RollRate : Inport  Port=7
  Clock1 : Clock
  Gaussian Noise Generator : commnoisgen2/Gaussian Noise Generator  m=NoiseMean  d=NoiseHeightVariance  s=41  Ts=Ts  frameBased=off  sampPerFrame=1  orient=off  outDataType=double
  Gaussian Noise Generator1 : commnoisgen2/Gaussian Noise Generator  m=NoiseMean  d=NoiseAngleVariance  s=41  Ts=Ts  frameBased=off  sampPerFrame=1  orient=off  outDataType=double
  Gaussian Noise Generator2 : commnoisgen2/Gaussian Noise Generator  m=NoiseMean  d=NoiseAngleRateVariance  s=41  Ts=Ts  frameBased=off  sampPerFrame=1  orient=off  outDataType=double
  Gaussian Noise Generator3 : commnoisgen2/Gaussian Noise Generator  m=NoiseMean  d=NoiseAngleVariance  s=41  Ts=Ts  frameBased=off  sampPerFrame=1  orient=off  outDataType=double
  Gaussian Noise Generator4 : commnoisgen2/Gaussian Noise Generator  m=NoiseMean  d=NoiseAngleRateVariance  s=41  Ts=Ts  frameBased=off  sampPerFrame=1  orient=off  outDataType=double
  Gaussian Noise Generator5 : commnoisgen2/Gaussian Noise Generator  m=NoiseMean  d=NoiseAngleVariance  s=41  Ts=Ts  frameBased=off  sampPerFrame=1  orient=off  outDataType=double
  Gaussian Noise Generator6 : commnoisgen2/Gaussian Noise Generator  m=NoiseMean  d=NoiseAngleRateVariance  s=41  Ts=Ts  frameBased=off  sampPerFrame=1  orient=off  outDataType=double
  Manual Switch{1,5..9} (6 alike) : ManualSwitch
  Manual Switch2 : ManualSwitch  CurrentSetting=0
  Manual Switch3 : ManualSwitch  CurrentSetting=0
  Manual Switch4 : ManualSwitch  CurrentSetting=0
  NoiseDelay{,1..6} (7 alike) : TransportDelay  DelayTime=NoiseDelay
  Pitch Sensor Filter : Subsystem
  Roll Sensor Filter1 : Subsystem
  Sum{1,3..5,7,9..10} (7 alike) : Sum  Inputs=++|
  Switch : Switch  Threshold=150
  To Workspace1 : ToWorkspace  VariableName=RollNoise  SampleTime=Ts  SaveFormat=Timeseries
  To Workspace2 : ToWorkspace  VariableName=PitchNoNoise  SampleTime=Ts  SaveFormat=Timeseries
  To Workspace3 : ToWorkspace  VariableName=PitchFilter  SampleTime=Ts  SaveFormat=Timeseries
  To Workspace5 : ToWorkspace  VariableName=PitchNoise  SampleTime=Ts  SaveFormat=Timeseries
  Transport Delay{,1..2,4..7} (7 alike) : TransportDelay  DelayTime=PropDelay
  Transport Delay3 : TransportDelay  DelayTime=200e-3
  Height1 : Outport
  Yaw1 : Outport  Port=2
  YawRate1 : Outport  Port=3
  Pitch1 : Outport  Port=4
  PitchRate1 : Outport  Port=5
  "Roll1 " : Outport  Port=6
  RollRate1 : Outport  Port=7
  wires:
  Sum1/1 -> Transport Delay/1
  Transport Delay7/1 -> Manual Switch8/1
  Sum3/1 -> Transport Delay1/1
  Transport Delay2/1 -> Manual Switch4/1
  Transport Delay/1 -> Manual Switch2/1
  Transport Delay5/1 -> Manual Switch6/1
  Manual Switch2/1 -> Height1/1
  Sum7/1 -> Transport Delay5/1
  Transport Delay4/1 -> Manual Switch5/1
  Gaussian Noise Generator2/1 -> NoiseDelay2/1
  Sum5/1 -> Transport Delay4/1
  Roll/1 -> Manual Switch7/2, Sum9/2
  Gaussian Noise Generator3/1 -> NoiseDelay3/1
  Gaussian Noise Generator/1 -> NoiseDelay/1
  Sum10/1 -> Transport Delay7/1
  Gaussian Noise Generator4/1 -> NoiseDelay4/1
  Sum9/1 -> Transport Delay6/1
  Gaussian Noise Generator1/1 -> NoiseDelay1/1
  PitchRate/1 -> Manual Switch6/2, Sum7/2
  Gaussian Noise Generator6/1 -> NoiseDelay6/1
  Height/1 -> Manual Switch2/2, Sum1/2
  Yaw/1 -> Manual Switch3/2, Sum3/2
  RollRate/1 -> Manual Switch8/2, Sum10/2
  Pitch/1 -> To Workspace2/1, Manual Switch5/2, Sum5/2
  Sum4/1 -> Transport Delay2/1
  Transport Delay1/1 -> Manual Switch3/1
  YawRate/1 -> Manual Switch4/2, Sum4/2
  Gaussian Noise Generator5/1 -> NoiseDelay5/1
  Manual Switch3/1 -> Yaw1/1
  Manual Switch4/1 -> YawRate1/1
  NoiseDelay/1 -> Sum1/1
  NoiseDelay1/1 -> Sum3/1
  NoiseDelay2/1 -> Sum4/1
  NoiseDelay3/1 -> Sum5/1
  NoiseDelay4/1 -> Sum7/1
  NoiseDelay5/1 -> Sum9/1
  NoiseDelay6/1 -> Sum10/1
  Transport Delay3/1 -> Switch/1
  Transport Delay6/1 -> Switch/3, Transport Delay3/1, To Workspace1/1
  Switch/1 -> Manual Switch7/1
  Clock1/1 -> Switch/2
  Manual Switch7/1 -> Roll Sensor Filter1/1(Roll Angle), Manual Switch1/2
  Manual Switch8/1 -> Roll Sensor Filter1/2(Roll Rate), RollRate1/1
  Roll Sensor Filter1/1(Roll Filtered) -> Manual Switch1/1
  Manual Switch1/1 -> "Roll1 "/1
  Manual Switch5/1 -> To Workspace5/1, Manual Switch9/2, Pitch Sensor Filter/1(Pitch Angle)
  Pitch Sensor Filter/1(Pitch Filtered) -> Manual Switch9/1
  Manual Switch9/1 -> To Workspace3/1, Pitch1/1
  Manual Switch6/1 -> Pitch Sensor Filter/2(Pitch Rate), PitchRate1/1

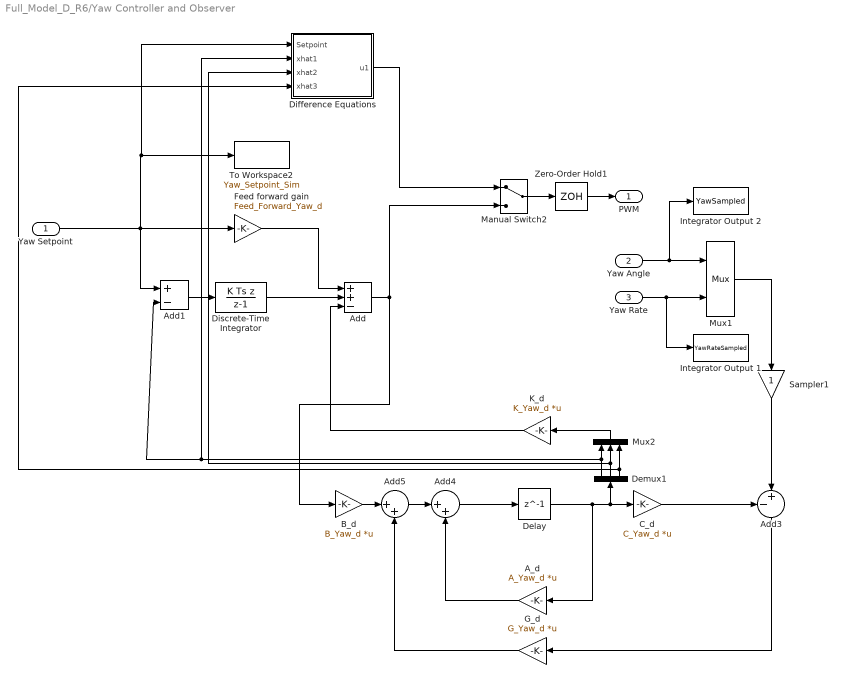
== system Full_Model_D_R6/Yaw Controller and Observer ==
  Yaw Setpoint : Inport
  Yaw Angle : Inport  Port=2
  Yaw Rate : Inport  Port=3
  A_d : Gain  Gain=A_Yaw_d  Multiplication=Matrix(K*u)  SampleTime=Ts
  Add : Sum  Inputs=++-
  Add1 : Sum  Inputs=+-
  Add3 : Sum  Inputs=-+|
  Add4 : Sum  Inputs=|++
  Add5 : Sum  Inputs=|++
  "B_d " : Gain  Gain=B_Yaw_d  Multiplication=Matrix(K*u)  SampleTime=Ts
  "C_d " : Gain  Gain=C_Yaw_d  Multiplication=Matrix(K*u)  SampleTime=Ts
  Delay : Delay  DelayLength=1  InitialCondition=0  SampleTime=Ts
  Demux1 : Demux  Outputs=3
  Difference Equations : Subsystem
  Discrete-Time Integrator : DiscreteIntegrator  IntegratorMethod=Integration: Backward Euler  gainval=-K_Yaw_i  SampleTime=Ts  ICPrevOutput=DiscIntNeverNeededParam  ICPrevScaledInput=DiscIntNeverNeededParam
  Feed forward gain : Gain  Gain=Feed_Forward_Yaw_d  SampleTime=Ts
  G_d : Gain  Gain=G_Yaw_d  Multiplication=Matrix(K*u)  SampleTime=Ts
  Integrator Output 1 : ToWorkspace  VariableName=YawRateSampled  SampleTime=Ts  SaveFormat=Timeseries
  Integrator Output 2 : ToWorkspace  VariableName=YawSampled  SampleTime=Ts  SaveFormat=Timeseries
  K_d : Gain  Gain=K_Yaw_d  Multiplication=Matrix(K*u)  SampleTime=Ts
  Manual Switch2 : ManualSwitch
  Mux1 : Mux  Inputs=2
      settings: DisplayOption=signals
  Mux2 : Mux  Inputs=3
  Sampler1 : Gain  SampleTime=Ts
  To Workspace2 : ToWorkspace  VariableName=Yaw_Setpoint_Sim  SampleTime=-1  SaveFormat=Timeseries
  Zero-Order Hold1 : ZeroOrderHold  SampleTime=Ts
  PWM : Outport
  wires:
  Yaw Setpoint/1 -> Add1/1, Difference Equations/1(Setpoint), To Workspace2/1, Feed forward gain/1
  Yaw Angle/1 -> Integrator Output 2/1, Mux1/1
  Yaw Rate/1 -> Integrator Output 1/1, Mux1/2
  Add1/1 -> Discrete-Time Integrator/1
  Demux1/1 -> Difference Equations/2(xhat1), Add1/2, Mux2/1
  Discrete-Time Integrator/1 -> Add/2
  Feed forward gain/1 -> Add/1
  Add/1 -> Manual Switch2/2, "B_d "/1
  Add3/1 -> G_d/1
  G_d/1 -> Add5/2
  Mux2/1 -> K_d/1
  Add5/1 -> Add4/1
  A_d/1 -> Add4/2
  Mux1/1 -> Sampler1/1
  Delay/1 -> Demux1/1, "C_d "/1, A_d/1
  Demux1/2 -> Mux2/2, Difference Equations/3(xhat2)
  Demux1/3 -> Difference Equations/4(xhat3), Mux2/3
  "B_d "/1 -> Add5/1
  "C_d "/1 -> Add3/1
  K_d/1 -> Add/3
  Add4/1 -> Delay/1
  Sampler1/1 -> Add3/2
  Difference Equations/1(u1) -> Manual Switch2/1
  Manual Switch2/1 -> Zero-Order Hold1/1
  Zero-Order Hold1/1 -> PWM/1

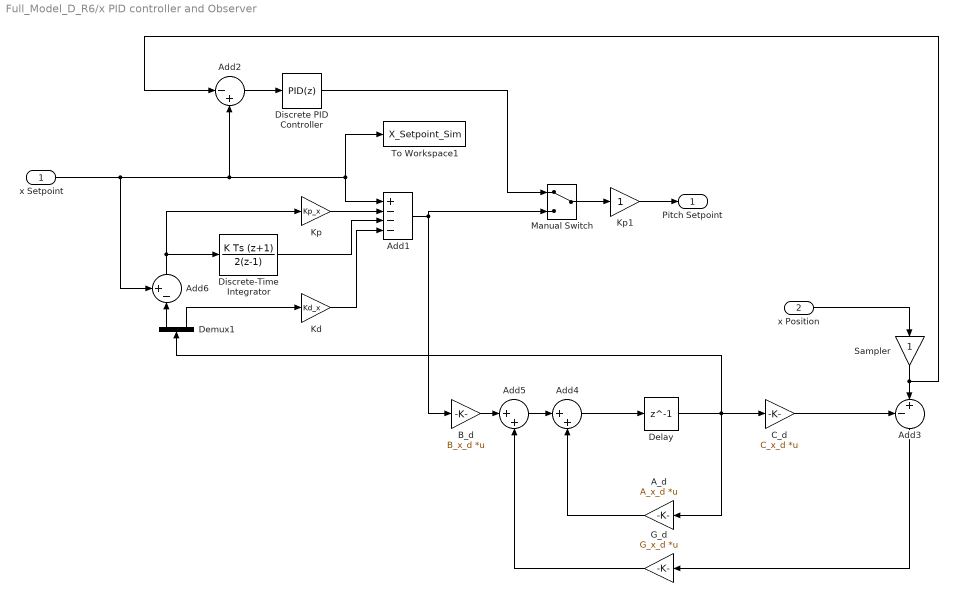
== system Full_Model_D_R6/x PID controller and Observer ==
  x Setpoint : Inport
  x Position : Inport  Port=2
  A_d : Gain  Gain=A_x_d  Multiplication=Matrix(K*u)  SampleTime=Ts2
  Add1 : Sum  Inputs=+---  SampleTime=Ts2
  Add2 : Sum  Inputs=|-+  SampleTime=Ts2
  Add3 : Sum  Inputs=-+|  SampleTime=Ts2
  Add4 : Sum  Inputs=|++  SampleTime=Ts2
  Add5 : Sum  Inputs=|++  SampleTime=Ts2
  Add6 : Sum  Inputs=+-|  SampleTime=Ts2
  "B_d " : Gain  Gain=B_x_d  Multiplication=Matrix(K*u)  SampleTime=Ts2
  "C_d " : Gain  Gain=C_x_d  Multiplication=Matrix(K*u)  SampleTime=Ts2
  Delay : Delay  DelayLength=1  InitialCondition=0  SampleTime=Ts2
  Demux1 : Demux  Outputs=2
  Discrete PID Controller : simulink/Continuous/PID Controller  Controller=PID  TimeDomain=Discrete-time  SampleTime=Ts2  IntegratorMethod=Forward Euler  FilterMethod=Forward Euler  Form=Parallel  P=Kp_x  I=Ki_x  D=Kd_x  N=100  InitialConditionSource=internal  InitialConditionForIntegrator=0  InitialConditionForFilter=0  ExternalReset=none  LimitOutput=off  UpperSaturationLimit=inf  LowerSaturationLimit=-inf  LinearizeAsGain=off  AntiWindupMode=none  Kb=1  TrackingMode=off  Kt=1  PParamMin=[]  PParamMax=[]  IParamMin=[]  IParamMax=[]  DParamMin=[]  DParamMax=[]  NParamMin=[]  NParamMax=[]  KbParamMin=[]  KbParamMax=[]  KtParamMin=[]  KtParamMax=[]  POutMin=[]  POutMax=[]  IOutMin=[]  IOutMax=[]  DOutMin=[]  DOutMax=[]  NOutMin=[]  NOutMax=[]  KbOutMin=[]  KbOutMax=[]  KtOutMin=[]  KtOutMax=[]  IntegratorOutMin=[]  IntegratorOutMax=[]  FilterOutMin=[]  FilterOutMax=[]  SumOutMin=[]  SumOutMax=[]  SumI1OutMin=[]  SumI1OutMax=[]  SumI2OutMin=[]  SumI2OutMax=[]  SumI3OutMin=[]  SumI3OutMax=[]  SumDOutMin=[]  SumDOutMax=[]  SaturationOutMin=[]  SaturationOutMax=[]  IntegratorContinuousStateAttributes=''  IntegratorStateMustResolveToSignalObject=off  IntegratorRTWStateStorageClass=Auto  FilterContinuousStateAttributes=''  FilterStateMustResolveToSignalObject=off  FilterRTWStateStorageClass=Auto
  Discrete-Time Integrator : DiscreteIntegrator  IntegratorMethod=Integration: Trapezoidal  gainval=Ki_x  SampleTime=Ts2  ICPrevOutput=DiscIntNeverNeededParam  ICPrevScaledInput=DiscIntNeverNeededParam
  G_d : Gain  Gain=G_x_d  Multiplication=Matrix(K*u)  SampleTime=Ts2
  Kd : Gain  Gain=Kd_x  SampleTime=Ts2
  Kp : Gain  Gain=Kp_x  SampleTime=Ts2
  Kp1 : Gain  SampleTime=Ts2
  Manual Switch : ManualSwitch
  Sampler : Gain  SampleTime=Ts2
  To Workspace1 : ToWorkspace  VariableName=X_Setpoint_Sim  SampleTime=Ts2  SaveFormat=Timeseries
  Pitch Setpoint : Outport
  wires:
  G_d/1 -> Add5/2
  A_d/1 -> Add4/2
  Kp/1 -> Add1/2
  Kd/1 -> Add1/4
  Add5/1 -> Add4/1
  x Setpoint/1 -> Add6/1, Add2/2, To Workspace1/1, Add1/1
  "C_d "/1 -> Add3/1
  Add4/1 -> Delay/1
  Delay/1 -> A_d/1, Demux1/1, "C_d "/1
  x Position/1 -> Sampler/1
  Demux1/2 -> Kd/1
  Add6/1 -> Kp/1, Discrete-Time Integrator/1
  Add3/1 -> G_d/1
  "B_d "/1 -> Add5/1
  Sampler/1 -> Add2/1, Add3/2
  Discrete-Time Integrator/1 -> Add1/3
  Discrete PID Controller/1 -> Manual Switch/1
  Manual Switch/1 -> Kp1/1
  Add2/1 -> Discrete PID Controller/1
  Demux1/1 -> Add6/2
  Add1/1 -> Manual Switch/2, "B_d "/1
  Kp1/1 -> Pitch Setpoint/1

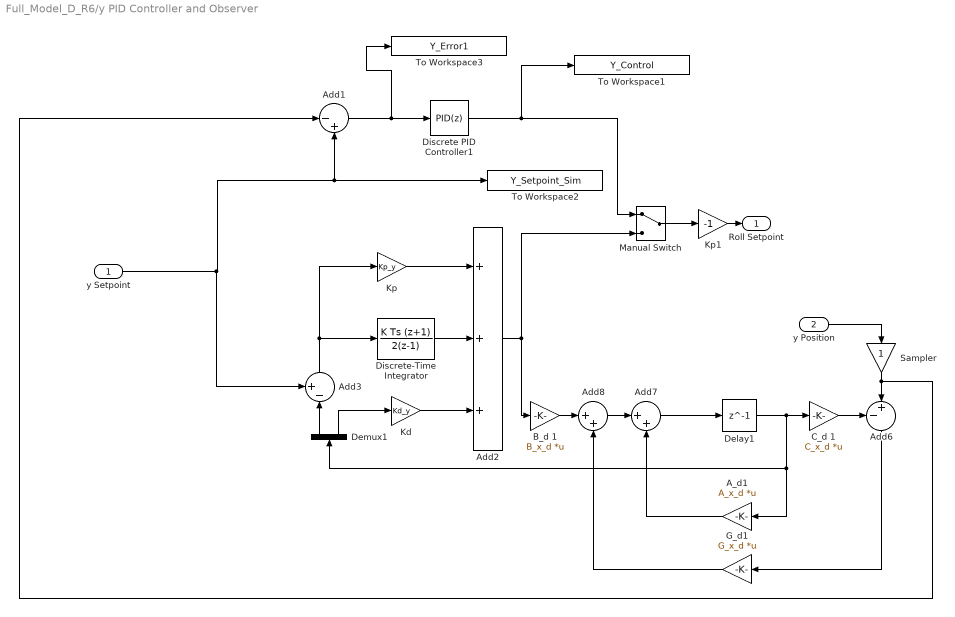
== system Full_Model_D_R6/y PID Controller and Observer ==
  y Setpoint : Inport
  y Position : Inport  Port=2
  A_d1 : Gain  Gain=A_x_d  Multiplication=Matrix(K*u)  SampleTime=Ts2
  Add1 : Sum  Inputs=|-+  SampleTime=Ts2
  Add2 : Sum  Inputs=+++  SampleTime=Ts2
  Add3 : Sum  Inputs=+-|  SampleTime=Ts2
  Add6 : Sum  Inputs=-+|
  Add7 : Sum  Inputs=|++  SampleTime=Ts2
  Add8 : Sum  Inputs=|++  SampleTime=Ts2
  B_d 1 : Gain  Gain=B_x_d  Multiplication=Matrix(K*u)  SampleTime=Ts2
  C_d 1 : Gain  Gain=C_x_d  Multiplication=Matrix(K*u)  SampleTime=Ts2
  Delay1 : Delay  DelayLength=1  InitialCondition=0  SampleTime=Ts2
  Demux1 : Demux  Outputs=2
  Discrete PID Controller1 : simulink/Continuous/PID Controller  Controller=PID  TimeDomain=Discrete-time  SampleTime=Ts2  IntegratorMethod=Forward Euler  FilterMethod=Forward Euler  Form=Parallel  P=Kp_y  I=Ki_y  D=Kd_y  N=100  InitialConditionSource=internal  InitialConditionForIntegrator=0  InitialConditionForFilter=0  ExternalReset=none  LimitOutput=off  UpperSaturationLimit=20  LowerSaturationLimit=-20  LinearizeAsGain=off  AntiWindupMode=none  Kb=1  TrackingMode=off  Kt=1  PParamMin=[]  PParamMax=[]  IParamMin=[]  IParamMax=[]  DParamMin=[]  DParamMax=[]  NParamMin=[]  NParamMax=[]  KbParamMin=[]  KbParamMax=[]  KtParamMin=[]  KtParamMax=[]  POutMin=[]  POutMax=[]  IOutMin=[]  IOutMax=[]  DOutMin=[]  DOutMax=[]  NOutMin=[]  NOutMax=[]  KbOutMin=[]  KbOutMax=[]  KtOutMin=[]  KtOutMax=[]  IntegratorOutMin=[]  IntegratorOutMax=[]  FilterOutMin=[]  FilterOutMax=[]  SumOutMin=[]  SumOutMax=[]  SumI1OutMin=[]  SumI1OutMax=[]  SumI2OutMin=[]  SumI2OutMax=[]  SumI3OutMin=[]  SumI3OutMax=[]  SumDOutMin=[]  SumDOutMax=[]  SaturationOutMin=[]  SaturationOutMax=[]  IntegratorContinuousStateAttributes=''  IntegratorStateMustResolveToSignalObject=off  IntegratorRTWStateStorageClass=Auto  FilterContinuousStateAttributes=''  FilterStateMustResolveToSignalObject=off  FilterRTWStateStorageClass=Auto
  Discrete-Time Integrator : DiscreteIntegrator  IntegratorMethod=Integration: Trapezoidal  gainval=Ki_y  SampleTime=Ts2  ICPrevOutput=DiscIntNeverNeededParam  ICPrevScaledInput=DiscIntNeverNeededParam
  G_d1 : Gain  Gain=G_x_d  Multiplication=Matrix(K*u)  SampleTime=Ts2
  Kd : Gain  Gain=Kd_y  SampleTime=Ts2
  Kp : Gain  Gain=Kp_y  SampleTime=Ts2
  Kp1 : Gain  Gain=-1  SampleTime=Ts2
  Manual Switch : ManualSwitch
  Sampler : Gain  SampleTime=Ts2
  To Workspace1 : ToWorkspace  VariableName=Y_Control  SampleTime=-1  SaveFormat=Timeseries
  To Workspace2 : ToWorkspace  VariableName=Y_Setpoint_Sim  SampleTime=-1  SaveFormat=Timeseries
  To Workspace3 : ToWorkspace  VariableName=Y_Error1  SampleTime=-1  SaveFormat=Timeseries
  Roll Setpoint : Outport
  wires:
  Add8/1 -> Add7/1
  y Setpoint/1 -> Add3/1, To Workspace2/1, Add1/2
  Kd/1 -> Add2/3
  y Position/1 -> Sampler/1
  Kp/1 -> Add2/1
  B_d 1/1 -> Add8/1
  Add7/1 -> Delay1/1
  C_d 1/1 -> Add6/1
  G_d1/1 -> Add8/2
  A_d1/1 -> Add7/2
  Add6/1 -> G_d1/1
  Add2/1 -> B_d 1/1, Manual Switch/2
  Delay1/1 -> C_d 1/1, Demux1/1, A_d1/1
  Demux1/2 -> Kd/1
  Add3/1 -> Discrete-Time Integrator/1, Kp/1
  Sampler/1 -> Add1/1, Add6/2
  Discrete-Time Integrator/1 -> Add2/2
  Manual Switch/1 -> Kp1/1
  Discrete PID Controller1/1 -> To Workspace1/1, Manual Switch/1
  Add1/1 -> To Workspace3/1, Discrete PID Controller1/1
  Demux1/1 -> Add3/2
  Kp1/1 -> Roll Setpoint/1

== system Full_Model_D_R6/Height Controller and Observer1/Difference Equations ==
  Setpoint : Inport
  xhat1 : Inport  Port=2
  xhat2 : Inport  Port=3
  xhat3 : Inport  Port=4
  Delay1 : Delay  DelayLength=1
  Mux : Mux  Inputs=5
  Mux3 : Mux  Inputs=3
  Roll Integator : Fcn  Expr=u(1) + ( -K_Height_i*Ts*( u(2)-u(3) ))  SampleTime=Ts
  Roll Regulator : Fcn  Expr=Feed_Forward_Height_d*u(1)+u(2)-K_Height_d(1)*u(3)-K_Height_d(2)*u(4)-K_Height_d(3)*u(5)  SampleTime=Ts
  u1 : Outport
  wires:
  Delay1/1 -> Mux3/1
  Mux/1 -> Roll Regulator/1
  xhat2/1 -> Mux/4
  xhat3/1 -> Mux/5
  xhat1/1 -> Mux/3, Mux3/3
  Setpoint/1 -> Mux3/2, Mux/1
  Roll Regulator/1 -> u1/1
  Roll Integator/1 -> Delay1/1, Mux/2  "v(k)"
  Mux3/1 -> Roll Integator/1

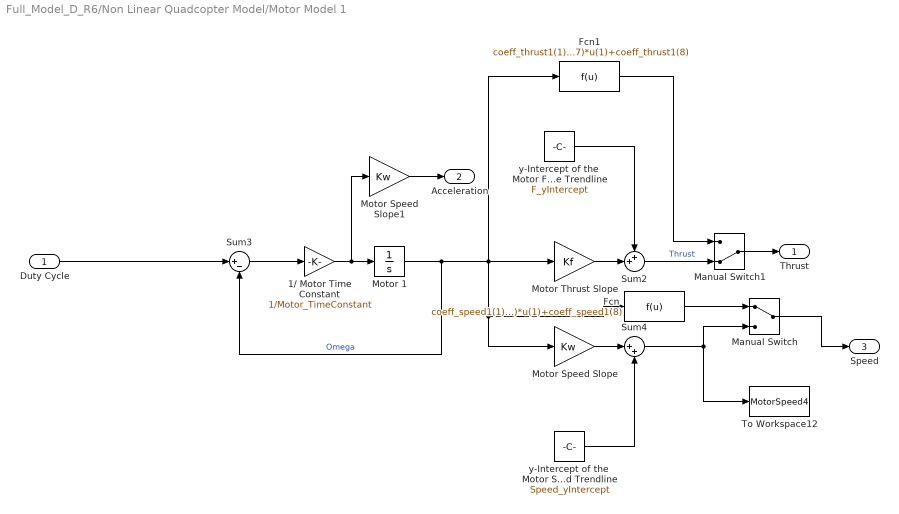
== system Full_Model_D_R6/Non Linear Quadcopter Model/Motor Model 1 ==
  Duty Cycle : Inport
  1/ Motor Time Constant : Gain  Gain=1/Motor_TimeConstant
  Fcn : Fcn  Expr=coeff_speed1(1)*u(1)^7 + coeff_speed1(2)*u(1)^6+coeff_speed1(3)*u(1)^5 + coeff_speed1(4)*u(1)^4+ coeff_speed1(5)*u(1)^3 +coeff_speed1(6)*u(1)^2+coeff_speed1(7)*u(1)+coeff_speed1(8)
  Fcn1 : Fcn  Expr=coeff_thrust1(1)*u(1)^7 + coeff_thrust1(2)*u(1)^6+coeff_thrust1(3)*u(1)^5 + coeff_thrust1(4)*u(1)^4+ coeff_thrust1(5)*u(1)^3 +coeff_thrust1(6)*u(1)^2+coeff_thrust1(7)*u(1)+coeff_thrust1(8)
  Manual Switch : ManualSwitch
  Manual Switch1 : ManualSwitch  CurrentSetting=0
  Motor 1 : Integrator  InitialCondition=omega_0  LimitOutput=on  LowerSaturationLimit=omega_Lim
  Motor Speed Slope : Gain  Gain=Kw
  Motor Speed Slope1 : Gain  Gain=Kw
  Motor Thrust Slope : Gain  Gain=Kf
  Sum2 : Sum  Inputs=++|
  Sum3 : Sum  Inputs=|+-
  Sum4 : Sum  Inputs=|++
  To Workspace12 : ToWorkspace  VariableName=MotorSpeed4  SampleTime=-1  SaveFormat=Timeseries
  y-Intercept of the  Motor Force Trendline : Constant  Value=F_yIntercept
  y-Intercept of the  Motor Speed Trendline : Constant  Value=Speed_yIntercept
  Thrust : Outport
  Acceleration : Outport  Port=2
  Speed : Outport  Port=3
  wires:
  Motor Thrust Slope/1 -> Sum2/2
  Motor 1/1 -> Sum3/2, Fcn1/1, Fcn/1, Motor Speed Slope/1, Motor Thrust Slope/1  "Omega"
  Duty Cycle/1 -> Sum3/1
  Sum3/1 -> 1/ Motor Time Constant/1
  1/ Motor Time Constant/1 -> Motor 1/1, Motor Speed Slope1/1
  Motor Speed Slope/1 -> Sum4/1
  Motor Speed Slope1/1 -> Acceleration/1
  Sum2/1 -> Manual Switch1/2  "Thrust"
  y-Intercept of the  Motor Force Trendline/1 -> Sum2/1
  y-Intercept of the  Motor Speed Trendline/1 -> Sum4/2
  Sum4/1 -> Manual Switch/2, To Workspace12/1
  Manual Switch/1 -> Speed/1
  Fcn/1 -> Manual Switch/1
  Manual Switch1/1 -> Thrust/1
  Fcn1/1 -> Manual Switch1/1

== system Full_Model_D_R6/Non Linear Quadcopter Model/Motor Model 2 ==
  Duty Cycle : Inport
  1/ Motor Time Constant : Gain  Gain=1/Motor_TimeConstant
  Fcn : Fcn  Expr=coeff_speed2(1)*u(1)^7 + coeff_speed2(2)*u(1)^6+coeff_speed2(3)*u(1)^5 + coeff_speed2(4)*u(1)^4+ coeff_speed2(5)*u(1)^3 +coeff_speed2(6)*u(1)^2+coeff_speed2(7)*u(1)+coeff_speed2(8)
  Fcn1 : Fcn  Expr=coeff_thrust2(1)*u(1)^7 + coeff_thrust2(2)*u(1)^6+coeff_thrust2(3)*u(1)^5 + coeff_thrust2(4)*u(1)^4+ coeff_thrust2(5)*u(1)^3 +coeff_thrust2(6)*u(1)^2+coeff_thrust2(7)*u(1)+coeff_thrust2(8)
  Manual Switch : ManualSwitch
  Manual Switch1 : ManualSwitch  CurrentSetting=0
  Motor 2 : Integrator  InitialCondition=omega_0  LimitOutput=on  LowerSaturationLimit=omega_Lim
  Motor Speed Slope : Gain  Gain=Kw
  Motor Speed Slope1 : Gain  Gain=Kw
  Motor Thrust Slope : Gain  Gain=Kf
  Sum2 : Sum  Inputs=++|
  Sum3 : Sum  Inputs=|+-
  Sum4 : Sum  Inputs=|++
  To Workspace9 : ToWorkspace  VariableName=MotorSpeed2  SampleTime=-1  SaveFormat=Timeseries
  y-Intercept of the  Motor Force Trendline : Constant  Value=F_yIntercept
  y-Intercept of the  Motor Speed Trendline : Constant  Value=Speed_yIntercept
  Thrust : Outport
  Acceleration : Outport  Port=2
  Speed : Outport  Port=3
  wires:
  Motor Thrust Slope/1 -> Sum2/2
  Motor 2/1 -> Sum3/2, Fcn1/1, Fcn/1, Motor Speed Slope/1, Motor Thrust Slope/1  "Omega"
  Duty Cycle/1 -> Sum3/1
  Sum3/1 -> 1/ Motor Time Constant/1
  1/ Motor Time Constant/1 -> Motor 2/1, Motor Speed Slope1/1
  Motor Speed Slope/1 -> Sum4/1
  Motor Speed Slope1/1 -> Acceleration/1
  Sum2/1 -> Manual Switch1/2  "Thrust"
  y-Intercept of the  Motor Force Trendline/1 -> Sum2/1
  Sum4/1 -> Manual Switch/2, To Workspace9/1  "Speed"
  y-Intercept of the  Motor Speed Trendline/1 -> Sum4/2
  Fcn/1 -> Manual Switch/1
  Manual Switch/1 -> Speed/1
  Manual Switch1/1 -> Thrust/1
  Fcn1/1 -> Manual Switch1/1

== system Full_Model_D_R6/Non Linear Quadcopter Model/Motor Model 3 ==
  Duty Cycle : Inport
  1/ Motor Time Constant : Gain  Gain=1/Motor_TimeConstant
  Fcn : Fcn  Expr=coeff_speed3(1)*u(1)^7 + coeff_speed3(2)*u(1)^6+coeff_speed3(3)*u(1)^5 + coeff_speed3(4)*u(1)^4+ coeff_speed3(5)*u(1)^3 +coeff_speed3(6)*u(1)^2+coeff_speed3(7)*u(1)+coeff_speed3(8)
  Fcn1 : Fcn  Expr=coeff_thrust3(1)*u(1)^7 + coeff_thrust3(2)*u(1)^6+coeff_thrust3(3)*u(1)^5 + coeff_thrust3(4)*u(1)^4+ coeff_thrust3(5)*u(1)^3 +coeff_thrust3(6)*u(1)^2+coeff_thrust3(7)*u(1)+coeff_thrust3(8)
  Manual Switch : ManualSwitch
  Manual Switch1 : ManualSwitch  CurrentSetting=0
  Motor 3 : Integrator  InitialCondition=omega_0  LimitOutput=on  LowerSaturationLimit=omega_Lim
  Motor Speed Slope : Gain  Gain=Kw
  Motor Speed Slope1 : Gain  Gain=Kw
  Motor Thrust Slope : Gain  Gain=Kf
  Sum2 : Sum  Inputs=++|
  Sum3 : Sum  Inputs=|+-
  Sum4 : Sum  Inputs=|++
  To Workspace11 : ToWorkspace  VariableName=MotorSpeed3  SampleTime=-1  SaveFormat=Timeseries
  y-Intercept of the  Motor Forc Trendline : Constant  Value=F_yIntercept
  y-Intercept of the  Motor Forc Trendline1 : Constant  Value=Speed_yIntercept
  Thrust : Outport
  Acceleration : Outport  Port=2
  Speed : Outport  Port=3
  wires:
  Motor Thrust Slope/1 -> Sum2/2  "Thrust"
  Motor 3/1 -> Sum3/2, Fcn/1, Motor Speed Slope/1, Fcn1/1, Motor Thrust Slope/1  "Omega"
  Duty Cycle/1 -> Sum3/1
  Sum3/1 -> 1/ Motor Time Constant/1
  1/ Motor Time Constant/1 -> Motor 3/1, Motor Speed Slope1/1
  Motor Speed Slope/1 -> Sum4/1
  Motor Speed Slope1/1 -> Acceleration/1
  y-Intercept of the  Motor Forc Trendline/1 -> Sum2/1
  y-Intercept of the  Motor Forc Trendline1/1 -> Sum4/2
  Sum2/1 -> Manual Switch1/2
  Sum4/1 -> Manual Switch/2, To Workspace11/1
  Manual Switch/1 -> Speed/1
  Fcn/1 -> Manual Switch/1
  Manual Switch1/1 -> Thrust/1
  Fcn1/1 -> Manual Switch1/1
